simulink library "gmt_Simulink"  (R2025a)
settings: Solver=ode23s  StartTime=0.0  StopTime=10.0  RelTol=1e-3
undefined symbols (not defined in the file or in its folder): graphMdl
settings Model: Creator=caksland  LastModifiedBy=jmp8430
settings OptimizationCC: ReuseModelBlockBuffer=off
settings RTWCC: GPUComputeCapability=3.5

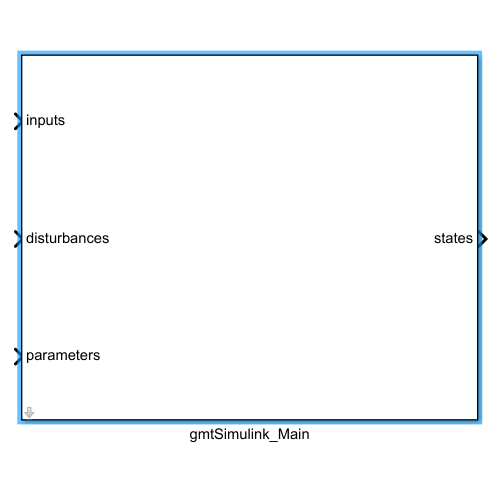
[thumbnail: Simulink's stored preview of the top-level diagram]
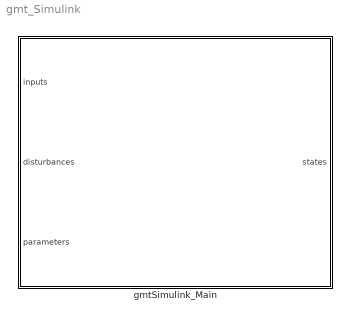
== system gmt_Simulink ==
  gmtSimulink_Main : Subsystem  mask{mdlName=graphMdl, x0=[300;300;300;300;6000;300;1500;300], x0_workspace_flg=off}
      mask prompts: mdlName "Model Name (must be object in working directory)"; x0 "Initial State (8):"; x0_workspace_flg "Pull initial conditions from workspace object?"
      settings: CopyFcn=set_param(gcb, 'LinkStatus', 'none');
      mask DialogControl Container7 Prompt: Description
      mask DialogControl Control6 Prompt: This Simulink block can be used to load and simulate a graph model generated with the graph modeling toolbox. The model name must be a gmt_Graph class or subclass object in the MATLAB  workspace. The initial conditions must be a column vector with the same number of rows as there are states. Users should verify solver using in simulations. ode23s has worked well for stiff dynamical system simulations.
      mask DialogControl DescGroupVar Prompt: States
      mask DialogControl States Prompt:
      | x1: CoolerLoad: Fluid Temperature
      | x3: EngineSplit: Junction Fluid Temperature
      | x5: HeatLoad: Fluid Temperature
      | x7: MainTank: Temperature
      | x8: MainTank: Mass
      | x12: RecirTank: Temperature
      | x13: RecirTank: Mass
      | x16: TankSplit: Junction Fluid Temperature
      mask DialogControl Container3 Prompt: Outputs
      mask DialogControl Container4 Prompt: Inputs
      mask DialogControl Inputs Prompt:
      | u6: MainTank Inlet Mass Flow 1
      | u7: MainTank Outlet Mass Flow 1
      | u8: RecirTank Inlet Mass Flow 1
      | u9: RecirTank Outlet Mass Flow 1
      mask DialogControl Container5 Prompt: Disturbances
      mask DialogControl Disturbances Prompt:
      | x2: CoolerLoad: Energy Applied
      | x6: HeatLoad: Energy Applied
      | x10: MainTank: Source Temperature
      mask DialogControl Container6 Prompt: Parameters
      mask DialogControl ParameterGroupVar Prompt: Model Configuration
      mask DialogControl mdlName_current Prompt: Current Model Loaded: graphMdl
      mask Display:
      | port_label('input', 1, 'inputs');
      | port_label('input', 2, 'disturbances');
      | port_label('input', 3, 'parameters');
      | port_label('output', 1, 'states');

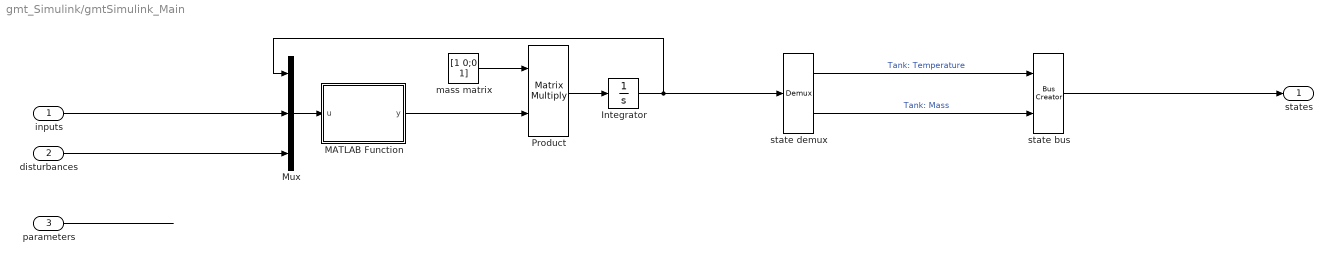
== system gmt_Simulink/gmtSimulink_Main ==
  inputs : Inport
  disturbances : Inport  Port=2
  parameters : Inport  Port=3
  Integrator : Integrator  InitialCondition=x0
  MATLAB Function : MATLAB Function  TreatAsAtomicUnit=on
  Mux : Mux  Inputs=3
  Product : Product  Multiplication=Matrix(*)
  mass matrix : Constant  Value=[1 0;0 1]
  state bus : BusCreator  Inputs=2
  state demux : Demux  Outputs=2
  states : Outport
  wires:
  Integrator/1 -> state demux/1, Mux/1
  parameters/1 -> ?
  Mux/1 -> MATLAB Function/1(u)
  mass matrix/1 -> Product/1
  MATLAB Function/1(y) -> Product/2
  Product/1 -> Integrator/1
  state bus/1 -> states/1
  inputs/1 -> Mux/2
  disturbances/1 -> Mux/3
  state demux/1 -> state bus/1  "Tank: Temperature"
  state demux/2 -> state bus/2  "Tank: Mass"

== matlab function gmt_Simulink/gmtSimulink_Main/MATLAB Function ==
  data: u input size=[5 1]; y output size=[2 1]
function y = fcn(u)
x1 = u(1);
x2 = u(2);
u1 = u(3);
u2 = u(4);
x4 = u(5);
cp_f = 3300;
x1_dot = -(cp_f*u2*x1 - cp_f*u1*x4 + cp_f*x1*(u1 - u2))/(cp_f*x2);
x2_dot = u1 - u2;
y = [x1_dot;x2_dot];
end
